simulink model "sliding_mode_ctrl"  (R2022b)
settings: Solver=ode1  StartTime=0.0  StopTime=10  FixedStep=0.001  RelTol=1e-3  EnableMultiTasking=on
undefined symbols (not defined in the file or in its folder): HIL
libraries: quarc_library x5, slpidlib x1
settings Model: SimulationMode=external  ExtModeTrigDuration=100001  Creator=smascaro  LastModifiedBy=willg
settings SolverCC: AlgebraicLoopSolver=TrustRegion  PositivePriorityOrder=on
settings DataIOCC: LimitDataPoints=on  SaveFormat=Array  SignalLoggingSaveFormat=ModelDataLogs  ReturnWorkspaceOutputs=off
settings OptimizationCC: ExpressionDepthLimit=2147483647  InitFltsAndDblsToZero=on
settings DebuggingCC: UnderspecifiedInitializationDetection=Classic  MergeDetectMultiDrivingBlocksExec=none  FcnCallInpInsideContextMsg=warning  UnconnectedInputMsg=warning  UnconnectedOutputMsg=warning  UnconnectedLineMsg=warning  AllowSymbolicDim=off  StateNameClashWarn=warning  SFUnexpectedBacktrackingDiag=warning  SFNoUnconditionalDefaultTransitionDiag=warning  SFExecutionAtInitializationDiag=none  SFMachineParentedDataDiag=warning  ArithmeticOperatorsInVariantConditions=warning
settings ModelReferenceCC: EnableRefExpFcnMdlSchedulingChecks=on  PropagateSignalLabelsOutOfModel=off
settings SFSimCC: SimUseLocalCustomCode=off  SimParseCustomCode=off  CustomCodeUndefinedFunction=UseInterfaceOnly
settings RTWCC: Description=QUARC Win64 Target Using Toolchain  SystemTargetFile=quarc_win64.tlc  TemplateMakefile=quarc_default_tmf  RTWUseLocalCustomCode=off  Toolchain=QUARC win64 | nmake (64-bit Windows)  BuildConfiguration=Faster Runs  DLArmComputeVersion=19.05
settings CodeAppCC: StateflowObjectComments=on
settings STFCustomTargetCC: ConcurrentExecutionCompliant=on  GRTInterface=on  UseToolchainInfoCompliant=on  SystemTargetFile=quarc_win64.tlc
settings GRTTargetCC: TargetLangStandard=C89/C90 (ANSI)  ParMdlRefBuildCompliant=off  CompOptLevelCompliant=off  CombineOutputUpdateFcns=off  MatFileLogging=off  CPPClassGenCompliant=off  GRTInterface=on  ExtMode=on  ExtModeMexFile=quarc_comm
settings ConfigComp: CovMetricSettings=dw  CovSaveCumulativeToWorkspaceVar=on  CovSaveSingleToWorkspaceVar=on  CovExternalEMLEnable=off

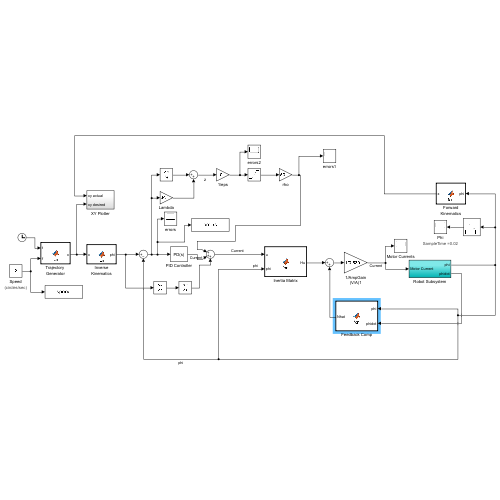
[thumbnail: Simulink's stored preview of the top-level diagram]
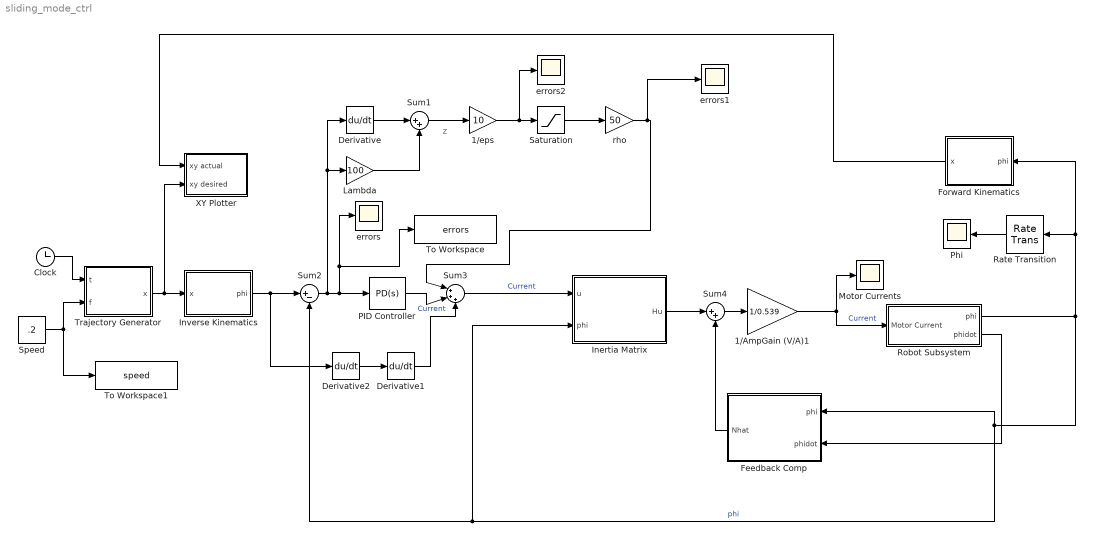
== system sliding_mode_ctrl ==
  note: z
  1/AmpGain (V/A)1 : Gain  Gain=1/0.539
  1/eps : Gain  Gain=10
  Clock : Clock
  Derivative : Derivative
  Derivative1 : Derivative
  Derivative2 : Derivative
  Feedback Comp : MATLAB Function  TreatAsAtomicUnit=on
  Forward Kinematics : MATLAB Function  TreatAsAtomicUnit=on
  Inertia Matrix : MATLAB Function  TreatAsAtomicUnit=on
  Inverse Kinematics : MATLAB Function  TreatAsAtomicUnit=on
  Lambda : Gain  Gain=100
  Motor Currents : Scope
  PID Controller : slpidlib/PID Controller  Controller=PD  Form=Parallel  TimeDomain=Continuous-time  UseExternalTs=off  SampleTime=-1  IntegratorMethod=Forward Euler  FilterMethod=Forward Euler  ControllerParametersSource=internal  P=1000  I=1  UseKiTs=off  D=39.8  N=100  UseFilter=on  TunerSelectOption=Transfer Function Based (PID Tuner App)  InitialConditionSource=internal  InitialConditionForIntegrator=0  InitialConditionForFilter=0  DifferentiatorICPrevScaledInput=0  ExternalReset=none  TrackingMode=off  Kt=1  LimitOutput=off  SatLimitsSource=internal  UpperSaturationLimit=inf  LowerSaturationLimit=-inf  LinearizeAsGain=on  AntiWindupMode=none  Kb=1  LimitIntegrator=off  UpperIntegratorSaturationLimit=inf  LowerIntegratorSaturationLimit=-inf  POutMin=[]  POutMax=[]  IOutMin=[]  IOutMax=[]  DOutMin=[]  DOutMax=[]  NOutMin=[]  NOutMax=[]  SumOutMin=[]  SumOutMax=[]  SaturationOutMin=[]  SaturationOutMax=[]  PParamMin=[]  PParamMax=[]  IParamMin=[]  IParamMax=[]  DParamMin=[]  DParamMax=[]  NParamMin=[]  NParamMax=[]  KbParamMin=[]  KbParamMax=[]  KtParamMin=[]  KtParamMax=[]  KbOutMin=[]  KbOutMax=[]  KtOutMin=[]  KtOutMax=[]  IntegratorOutMin=[]  IntegratorOutMax=[]  FilterOutMin=[]  FilterOutMax=[]  SumI1OutMin=[]  SumI1OutMax=[]  SumI2OutMin=[]  SumI2OutMax=[]  SumI3OutMin=[]  SumI3OutMax=[]  SumI4OutMin=[]  SumI4OutMax=[]  SumDOutMin=[]  SumDOutMax=[]  DifferentiatorOutMin=[]  DifferentiatorOutMax=[]  FilterDiffOutCoefMin=[]  FilterDiffOutCoefMax=[]  ReciprocalOutMin=[]  ReciprocalOutMax=[]  SumDenOutMin=[]  SumDenOutMax=[]  SumNumOutMin=[]  SumNumOutMax=[]  DivideOutMin=[]  DivideOutMax=[]  UdiffTsProdOutMin=[]  UdiffTsProdOutMax=[]  NTsProdOutMin=[]  NTsProdOutMax=[]  UintegralTsProdOutMin=[]  UintegralTsProdOutMax=[]  UngainTsProdOutMin=[]  UngainTsProdOutMax=[]  ClampingZeroOutDataTypeStr=Inherit: Inherit via back propagation  ClampingZeroOutMin=[]  ClampingZeroOutMax=[]  FilterDenConstantOutDataTypeStr=Inherit: Inherit via back propagation  FilterDenConstantOutMin=[]  FilterDenConstantOutMax=[]  PCopyOutDataTypeStr=Inherit: Inherit via back propagation  PCopyOutMin=[]  PCopyOutMax=[]  NCopyOutDataTypeStr=Inherit: Inherit via back propagation  NCopyOutMin=[]  NCopyOutMax=[]  IntegratorContinuousStateAttributes=''  IntegratorStateMustResolveToSignalObject=off  IntegratorRTWStateStorageClass=Auto  FilterContinuousStateAttributes=''  FilterStateMustResolveToSignalObject=off  FilterRTWStateStorageClass=Auto  ParallelPVariant=InternalParameters  IdealPVariant=Disabled  IVariant=Disabled  DVariant=InternalParameters  IntegratorVariant=Disabled  SatVariant=Disabled  AWVariant=Disabled  PCopyVariant=Disabled  TRVariant=Disabled  FdbkBlocksVariant=Forward  IdealPFdbkVariant=Disabled  SatFdbkVariant=Disabled  DerivativeFilterVariant=ContFilter  NVariant=InternalParameters  NCopyVariant=Disabled  FilterICVariant=InternalICsFilter  IntegratorICVariant=Disabled  ExternalResetVariant=Disabled  TRSumVariant=Passthrough  SumFdbkVariant=Disabled  SumVariant=Sum_PD  TsampFilterVariant=InternalTs  TsampNgainVariant=Passthrough  TsampIntegralVariant=Disabled_SignalSpec  ExternalSaturationOutDataTypeStr=Inherit: Same as second input
  Phi : Scope
      settings: AttributesFormatString=SampleTime =%<SampleTime>
  Rate Transition : RateTransition  OutPortSampleTimeOpt=Inherit  OutPortSampleTimeMultiple=10  OutPortSampleTime=0.05
  Robot Subsystem : Subsystem
  Saturation : Saturate  UpperLimit=.2  LowerLimit=-.2
  Speed : Constant  Value=.2
      settings: AttributesFormatString=(circles/sec)
  Sum1 : Sum  Inputs=|++
  Sum2 : Sum  Inputs=|+-
  Sum3 : Sum  Inputs=|+++
  Sum4 : Sum  Inputs=|++
  To Workspace : ToWorkspace  VariableName=errors  SaveFormat=Timeseries  SampleTime=-1
  To Workspace1 : ToWorkspace  VariableName=speed  SampleTime=-1
  Trajectory Generator : MATLAB Function  TreatAsAtomicUnit=on
  XY Plotter : Subsystem
  errors : Scope
  errors1 : Scope
  errors2 : Scope
  rho : Gain  Gain=50
  wires:
  Trajectory Generator/1(x) -> Inverse Kinematics/1(x), XY Plotter/2(xy desired)
  Clock/1 -> Trajectory Generator/1(t)
  Speed/1 -> Trajectory Generator/2(f), To Workspace1/1
  Forward Kinematics/1(x) -> XY Plotter/1(xy actual)
  Rate Transition/1 -> Phi/1
  PID Controller/1 -> Sum3/2  "Current"
  Feedback Comp/1(Nhat) -> Sum4/2
  1/AmpGain (V/A)1/1 -> Motor Currents/1, Robot Subsystem/1(Motor Current)  "Current"
  Derivative1/1 -> Sum3/3
  Derivative2/1 -> Derivative1/1
  Sum4/1 -> 1/AmpGain (V/A)1/1
  Inertia Matrix/1(Hu) -> Sum4/1
  Robot Subsystem/1(phi) -> Inertia Matrix/2(phi), Sum2/2, Feedback Comp/1(phi), Forward Kinematics/1(phi), Rate Transition/1  "phi"
  Sum3/1 -> Inertia Matrix/1(u)  "Current"
  Inverse Kinematics/1(phi) -> Sum2/1, Derivative2/1
  Robot Subsystem/2(phidot) -> Feedback Comp/2(phidot)
  Saturation/1 -> rho/1
  Derivative/1 -> Sum1/1
  rho/1 -> errors1/1, Sum3/1
  1/eps/1 -> errors2/1, Saturation/1
  Sum1/1 -> 1/eps/1
  Sum2/1 -> Lambda/1, Derivative/1, To Workspace/1, errors/1, PID Controller/1
  Lambda/1 -> Sum1/2

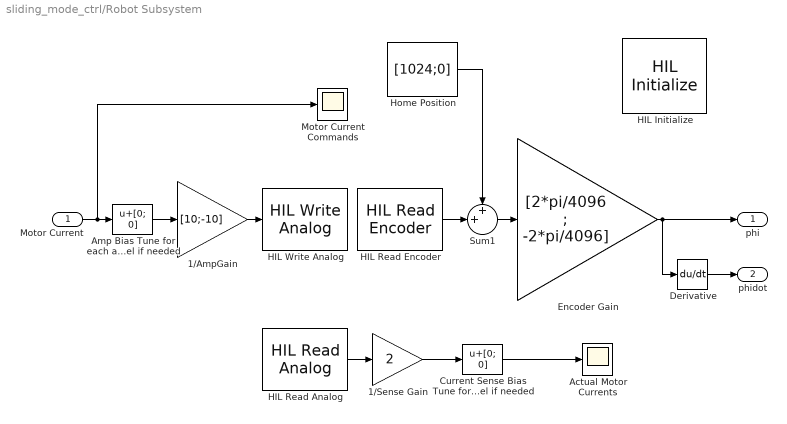
== system sliding_mode_ctrl/Robot Subsystem ==
  Motor Current : Inport
  1/AmpGain : Gain  Gain=[10;-10]
  1/Sense Gain : Gain  Gain=2
  Actual Motor Currents : Scope
  Amp Bias Tune for each amp/channel if needed : Bias  Bias=[0; 0]  SaturateOnIntegerOverflow=off
  Current Sense Bias Tune for each amp/channel if needed : Bias  Bias=[0; 0]  SaturateOnIntegerOverflow=off
  Derivative : Derivative
  Encoder Gain : Gain  Gain=[2*pi/4096 ; -2*pi/4096]
  HIL Initialize : quarc_library/Data Acquisition/Generic/Configuration/HIL Initialize  object_name=HIL-1  board_type=q8_usb  board_number=0  board_options=update_rate=normal  exclusive=off  active=off  hardware_clocks=[0:2]  clock_modes=[]  initial_clock_frequencies=[]  set_clock_params_at_start=off  set_clock_params_at_switch_in=off  set_clock_frequencies_at_start=off  set_clock_frequencies_at_switch_in=off  analog_input_channels=[0:7]  analog_input_configurations=[]  analog_input_maximums=10  analog_input_minimums=-10  set_analog_input_params_at_start=on  set_analog_input_params_at_switch_in=off  analog_output_channels=[0:7]  analog_output_maximums=10  analog_output_minimums=-10  initial_analog_outputs=[0]  final_analog_outputs=[0]  watchdog_analog_outputs=0  set_analog_output_params_at_start=on  set_analog_output_params_at_switch_in=off  set_analog_outputs_at_start=on  set_analog_outputs_at_switch_in=off  set_analog_outputs_at_terminate=on  set_analog_outputs_at_switch_out=off  set_analog_outputs_on_watchdog=off  digital_input_channels=[]  digital_output_channels=[]  digital_output_configuration=[]  initial_digital_outputs=[1]  final_digital_outputs=[1]  watchdog_digital_outputs=[1]  set_digital_output_params_at_start=off  set_digital_output_params_at_switch_in=off  set_digital_outputs_at_start=on  set_digital_outputs_at_switch_in=off  set_digital_outputs_at_terminate=on  set_digital_outputs_at_switch_out=off  set_digital_outputs_on_watchdog=off  encoder_channels=[0:7]  quadrature=[4]  encoder_filter_frequency=[]  initial_encoder_counts=[0]  set_encoder_params_at_start=on  set_encoder_params_at_switch_in=off  set_encoder_counts_at_start=on  set_encoder_counts_at_switch_in=off  pwm_channels=[0:7]  pwm_modes=0  pwm_frequency=99.532799999999995e6/4095  pwm_configuration=[0]  pwm_alignment=[0]  pwm_polarity=[1]  pwm_leading_deadband=[0]  pwm_trailing_deadband=[0]  initial_pwm_outputs=[0]  final_pwm_outputs=[0]  watchdog_pwm_outputs=[0]  set_pwm_params_at_start=on  set_pwm_params_at_switch_in=off  set_pwm_outputs_at_start=on  set_pwm_outputs_at_switch_in=off  set_pwm_outputs_at_terminate=on  set_pwm_outputs_at_switch_out=off  set_pwm_outputs_on_watchdog=off  other_output_channels=[]  initial_other_outputs=[]  final_other_outputs=[]  watchdog_other_outputs=[]  set_other_outputs_at_start=off  set_other_outputs_at_switch_in=off  set_other_outputs_at_terminate=off  set_other_outputs_at_switch_out=off  set_other_outputs_on_watchdog=off
  HIL Read Analog : quarc_library/Data Acquisition/Generic/Immediate I//O/HIL Read Analog  object_name=HIL-1  channels=[0;1]  sample_time=qc_get_step_size  active=on  vector_output=on
  HIL Read Encoder : quarc_library/Data Acquisition/Generic/Immediate I//O/HIL Read Encoder  object_name=HIL-1  channels=[0:1]  sample_time=qc_get_step_size  active=on  vector_output=on  data_type_mode=Inherit via back propagation  data_type=double
  HIL Write Analog : quarc_library/Data Acquisition/Generic/Immediate I//O/HIL Write Analog  object_name=HIL-1  channels=[0:1]  sample_time=-1  active=off  vector_input=on
  Home Position : Constant  Value=[1024;0]  VectorParams1D=off
  Motor Current Commands : Scope
  Sum1 : Sum  Inputs=++|
  phi : Outport  VectorParamsAs1DForOutWhenUnconnected=off
  phidot : Outport  Port=2  VectorParamsAs1DForOutWhenUnconnected=off
  wires:
  1/AmpGain/1 -> HIL Write Analog/1
  Encoder Gain/1 -> phi/1, Derivative/1
  Derivative/1 -> phidot/1
  HIL Read Analog/1 -> 1/Sense Gain/1
  Motor Current/1 -> Amp Bias Tune for each amp/channel if needed/1, Motor Current Commands/1
  Amp Bias Tune for each amp/channel if needed/1 -> 1/AmpGain/1
  Home Position/1 -> Sum1/1
  HIL Read Encoder/1 -> Sum1/2
  Sum1/1 -> Encoder Gain/1
  1/Sense Gain/1 -> Current Sense Bias Tune for each amp/channel if needed/1
  Current Sense Bias Tune for each amp/channel if needed/1 -> Actual Motor Currents/1

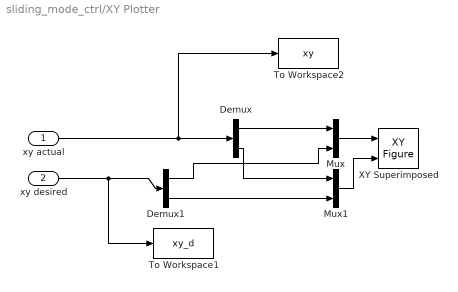
== system sliding_mode_ctrl/XY Plotter ==
  xy actual : Inport
  xy desired : Inport  Port=2
  Demux : Demux  Outputs=2
  Demux1 : Demux  Outputs=2
  Mux : Mux  Inputs=2
  Mux1 : Mux  Inputs=2
  To Workspace1 : ToWorkspace  VariableName=xy_d  SampleTime=-1
  To Workspace2 : ToWorkspace  VariableName=xy  SampleTime=-1
  XY Superimposed : quarc_library/Sinks/Figures/XY Figure  figure_mode=Use figure window  figure_tag=figure1  axes_tag=axes1  plot_mode=Time-based  minimum_x=0  maximum_x=.3  minimum_y=0  maximum_y=.2  buffer_size=10000  update_rate=100  initial_position="825           185         623.2         411.2"  initial_visibility=off  sample_time=-1
  wires:
  Demux/2 -> Mux1/1
  Mux1/1 -> XY Superimposed/2
  Mux/1 -> XY Superimposed/1
  Demux/1 -> Mux/1
  xy desired/1 -> Demux1/1, To Workspace1/1
  Demux1/1 -> Mux/2
  Demux1/2 -> Mux1/2
  xy actual/1 -> Demux/1, To Workspace2/1

== matlab function sliding_mode_ctrl/Forward Kinematics ==
  settings: fimath=|
      | fimath(...
      | 'RoundMode', 'floor',...
      | 'OverflowMode', 'wrap',...
      | 'ProductMode', 'KeepLSB', 'ProductWordLength', 32,...
      | 'SumMode', 'KeepLSB', 'SumWordLength', 32,...
      | 'CastBeforeSum', false)
  data: x output; phi input
function x = fcn(phi)
% This block supports an embeddable subset of the MATLAB language.
% See the help menu for details. 
a1=.15;
a2=.15;
x = [0;0];
x(1) = a1*cos(phi(1))+a2*cos(phi(2));
x(2) = a1*sin(phi(1))+a2*sin(phi(2));

== matlab function sliding_mode_ctrl/Feedback Comp ==
  settings: fimath=|
      | fimath(...
      | 'RoundMode', 'floor',...
      | 'OverflowMode', 'wrap',...
      | 'ProductMode', 'KeepLSB', 'ProductWordLength', 32,...
      | 'SumMode', 'KeepLSB', 'SumWordLength', 32,...
      | 'CastBeforeSum', false)
  data: Nhat output; phi input; phidot input
function Nhat = fcn(phi, phidot)
% Feedback Comp 

a1 = 0.15;  % link 1 length
a2 = 0.15;  % link 2 length
m1 = 0.092;  % link 1 mass  
m2 = 0.077; % link 2 mas
r01 = 0.062; % link 1 center of mass
r12 = 0.036; % link 2 COM
I1 = 0.64e-3;  % link 1 inertia
I2 = 0.30e-3;  % link 2 inertia
Jm1 = 0.65e-6; % motor inertias
Jm2 = 0.65e-6;
b1 = 3.1e-6; % viscous damping constants
b2 = 3.1e-6;
c1 = 0.0001; % coulomb friction constants
c2 = 0.0001;
g = 9.8; % gravitational constant
N1 = 70; % gear ratios
N2 = 70;

h = a1*r12*m2*sin(phi(2)-phi(1));
G1 = (r01*m1+a1*m2)*g*cos(phi(1));
G2 = r12*m2*g*cos(phi(2));
F1 = N1^2*b1*phidot(1) + N1*c1*sign(phidot(1));
F2 = N2^2*b2*phidot(2) + N2*c2*sign(phidot(2));

V = [0 -h ;h 0]*[phidot(1)^2;phidot(2)^2]; % centr torques
G = [G1;G2]; % gravity torques
F = [F1;F2]; % frictional torques

Nhat = V + G + F;

== matlab function sliding_mode_ctrl/Inertia Matrix ==
  settings: fimath=|
      | fimath(...
      | 'RoundMode', 'floor',...
      | 'OverflowMode', 'wrap',...
      | 'ProductMode', 'KeepLSB', 'ProductWordLength', 32,...
      | 'SumMode', 'KeepLSB', 'SumWordLength', 32,...
      | 'CastBeforeSum', false)
  data: u input; Hu output; phi input
function Hu = fcn(u, phi)
% Inertia Matrix. 

a1 = 0.15;  % link 1 length
a2 = 0.15;  % link 2 length
m1 = 0.092;  % link 1 mass  
m2 = 0.077; % link 2 mas
r01 = 0.062; % link 1 center of mass
r12 = 0.036; % link 2 COM
I1 = 0.64e-3;  % link 1 inertia
I2 = 0.30e-3;  % link 2 inertia
Jm1 = 0.65e-6; % motor inertias
Jm2 = 0.65e-6;
b1 = 3.1e-6; % viscous damping constants
b2 = 3.1e-6;
c1 = 0.0001; % coulomb friction constants
c2 = 0.0001;
g = 9.8; % gravitational constant
N1 = 70; % gear ratios
N2 = 70;

H11 = N1^2*Jm1 + I1 + m2*a1^2;
H12 = a1*r12*m2*cos(phi(2)-phi(1));
H21 = H12;
H22 = N2^2*Jm2 + I2;

H = [H11 H12; H21 H22]; % inertia matrix

Hu = H*u;

== matlab function sliding_mode_ctrl/Trajectory Generator ==
  settings: fimath=|
      | fimath(...
      | 'RoundMode', 'floor',...
      | 'OverflowMode', 'wrap',...
      | 'ProductMode', 'KeepLSB', 'ProductWordLength', 32,...
      | 'SumMode', 'KeepLSB', 'SumWordLength', 32,...
      | 'CastBeforeSum', false)
  data: x output; t input; f input
function x = fcn(t,f)
% This block supports an embeddable subset of the MATLAB language.
% See the help menu for details. 
x = [0;0];

if t<1 % move robot smoothly from home position @ x=[1.5,1.5] to point on circle @ x=[0.2,0.1]
        x(1) = 0.15 + 0.025*(1 - cos(pi*t));
        x(2) = 0.15 - 0.025*(1 - cos(pi*t));
elseif t<1.5  % accelerate into circling trajectory
    x(1) = 0.075*cos(2*pi*f*(t-1)^2) + 0.125;
    x(2) = 0.075*sin(2*pi*f*(t-1)^2) + 0.1;
else  % constant speed circling of radius 0.075 about x=[0.125,0.1]
    x(1) = 0.075*cos(2*pi*f*(t-1.25)) + 0.125;
    x(2) = 0.075*sin(2*pi*f*(t-1.25)) + 0.1;
end

== matlab function sliding_mode_ctrl/Inverse Kinematics ==
  settings: fimath=|
      | fimath(...
      | 'RoundMode', 'floor',...
      | 'OverflowMode', 'wrap',...
      | 'ProductMode', 'KeepLSB', 'ProductWordLength', 32,...
      | 'SumMode', 'KeepLSB', 'SumWordLength', 32,...
      | 'CastBeforeSum', false)
  data: x input; phi output
function phi = fcn(x)
% This block supports an embeddable subset of the MATLAB language.
% See the help menu for details. 
a1=0.15;
a2=0.15;
Jt = [1 0; -1 1]; % belt drive Jabobian
theta = [0;0];
theta(2) = -2*atan(sqrt(((a1+a2)^2-(x(1)^2+x(2)^2))/((x(1)^2+x(2)^2)-(a1-a2)^2)));
theta(1) = atan2(x(2),x(1))-atan2(a2*sin(theta(2)),a1+a2*cos(theta(2)));
phi = inv(Jt)*theta; % convert to absolute joint angles
